simulink model "TP1_Simulink"  (R2021a)
settings: Solver=ode4  StartTime=0.0  StopTime=3000  FixedStep=1  RelTol=1e-3
values from neighbouring files (symbols this model uses):
  h0 = h0_vec(i)    [TP1.m]    (also in TP1_ParteMatlab.m = 0.45)
  u0 = Qi / (A_sal * sqrt(2 * g * h0))    [TP1.m]    (also in TP1_ParteMatlab.m)
libraries: cstblocks x2
settings Model: Creator=aghersin  LastModifiedBy=faust
settings SolverCC: AlgebraicLoopSolver=TrustRegion
settings DataIOCC: ReturnWorkspaceOutputs=off
settings OptimizationCC: LifeSpan=inf
settings DebuggingCC: SFExecutionAtInitializationDiag=none  SFMachineParentedDataDiag=warning  ArithmeticOperatorsInVariantConditions=warning
settings SFSimCC: SimUseLocalCustomCode=off  CustomCodeUndefinedFunction=UseInterfaceOnly
settings RTWCC: RTWUseLocalCustomCode=off
settings CodeAppCC: StateflowObjectComments=on

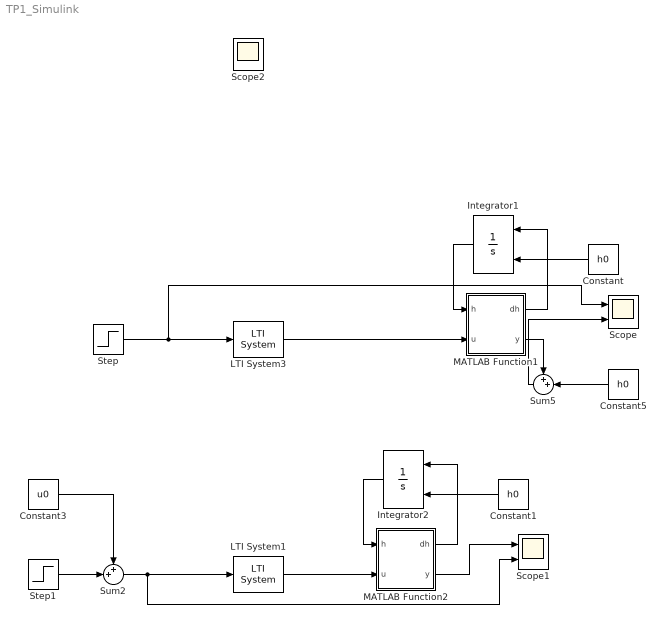
== system TP1_Simulink ==
  Constant : Constant  Value=h0
  Constant1 : Constant  Value=h0
  Constant3 : Constant  Value=u0
  Constant5 : Constant  Value=h0
  Integrator1 : Integrator  InitialConditionSource=external
  Integrator2 : Integrator  InitialConditionSource=external
  LTI System1 : cstblocks/LTI System  sys=1  IC=[]
  LTI System3 : cstblocks/LTI System  sys=1  IC=[]
  MATLAB Function1 : MATLAB Function  TreatAsAtomicUnit=on
  MATLAB Function2 : MATLAB Function  TreatAsAtomicUnit=on
  Scope : Scope  NumInputPorts=2
  Scope1 : Scope  NumInputPorts=2
  Step : Step  Time=10  After=u0 * 0.1  SampleTime=0
  Step1 : Step  Time=10  After=u0 * 0.1  SampleTime=0
  Sum2 : Sum  Inputs=++|
  Sum5 : Sum  Inputs=++|
  Scope2 : Scope
  wires:
  Integrator1/1 -> MATLAB Function1/1(h)
  MATLAB Function1/1(dh) -> Integrator1/1
  MATLAB Function1/2(y) -> Sum5/1
  Constant5/1 -> Sum5/2
  Step/1 -> Scope/1, LTI System3/1
  LTI System3/1 -> MATLAB Function1/2(u)
  Constant/1 -> Integrator1/2
  Constant3/1 -> Sum2/1
  Step1/1 -> Sum2/2
  Integrator2/1 -> MATLAB Function2/1(h)
  Constant1/1 -> Integrator2/2
  MATLAB Function2/2(y) -> Scope1/1
  MATLAB Function2/1(dh) -> Integrator2/1
  Sum2/1 -> LTI System1/1, Scope1/2
  LTI System1/1 -> MATLAB Function2/2(u)
  Sum5/1 -> Scope/2

== matlab function TP1_Simulink/MATLAB Function2 ==
  data: h input; u input; dh output; y output
function [dh,y] = fcn(h,u)
g = 9.8;        %En metros sobre segundo cuadrado
L = 0.9;        %En metros
L_h = 0.4;      %En metros
L_l = 0.1;      %En metros
Qi = 0.0001333; %Metros cubicos por segundo
d2 = 10.65e-3;
A_sal = pi * (d2 / 2)^2;
L1 = L_l /(L_h - L_l) * L;
dh = 3 * L1^2 * (Qi - A_sal * u * sqrt(2 * g * h))/(L_l^2 * (3 * h^2 + 6 * L1 * h + 3 * L1^2)) ;
y = h;

== matlab function TP1_Simulink/MATLAB Function1 ==
  data: h input; u input; dh output; y output
function [dh,y] = fcn(h,u)
dh = -0.0024 * h - 0.0042 * u;
y = h;
